simulink model "pendenc"  (Simulink 6.2)
settings: Solver=ode45  StartTime=0.0  StopTime=100.0  RelTol=1e-4
libraries: cstblocks x10, simulink x6
settings Model: Creator=mbarton  LastModifiedBy=mbarton  ExtModeTrigMode=oneshot  ExtModeArmWhenConnect=off  ExtModeAutoUpdateStatusClock=off  BufferReuse=off
settings DataIOCC: LimitDataPoints=off
settings OptimizationCC: BlockReduction=off  BooleanDataType=off  InlineParams=on  InlineInvariantSignals=on  BufferReuse=off
settings HardwareCC: TargetUnknown=on

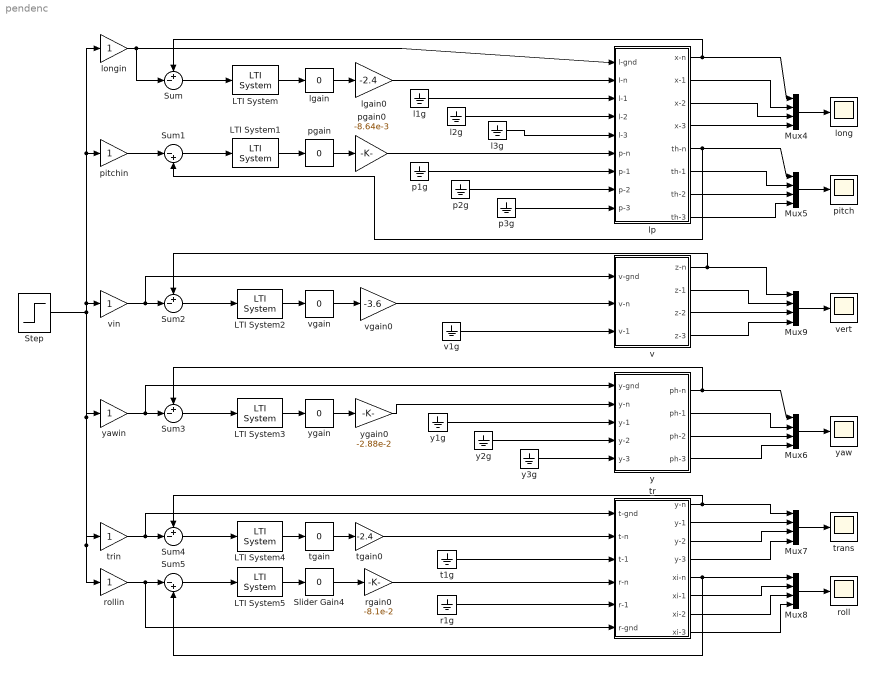
== system pendenc ==
  LTI System : cstblocks/LTI System  sys=ldamp  IC=[]
  LTI System1 : cstblocks/LTI System  sys=pdamp  IC=[]
  LTI System2 : cstblocks/LTI System  sys=vdamp  IC=[]
  LTI System3 : cstblocks/LTI System  sys=ydamp  IC=[]
  LTI System4 : cstblocks/LTI System  sys=tdamp  IC=[]
  LTI System5 : cstblocks/LTI System  sys=rdamp  IC=[]
  Mux{4..9} (6 alike) : Mux
  Slider Gain4 : simulink/Math Operations/Slider Gain  low=0  gain=0  high=2
  Step : Step  Before=1  After=0  SampleTime=0
  Sum{,2..4} (4 alike) : Sum  Inputs=+-|  InputSameDT=on
  Sum1 : Sum  Inputs=|-+  InputSameDT=on
  Sum5 : Sum  Inputs=|-+  InputSameDT=on
  l1g : Ground
  l2g : Ground
  l3g : Ground
  lgain : simulink/Math Operations/Slider Gain  low=0  gain=0  high=2
  lgain0 : Gain  Gain=-2.4
  long : Scope
  longin : Gain
  lp : Subsystem
  p1g : Ground
  p2g : Ground
  p3g : Ground
  pgain : simulink/Math Operations/Slider Gain  low=0  gain=0  high=2
  pgain0 : Gain  Gain=-8.64e-3
  pitch : Scope
  pitchin : Gain
  r1g : Ground
  rgain0 : Gain  Gain=-8.1e-2
  roll : Scope
      settings: YMin=-2  YMax=2
  rollin : Gain
  t1g : Ground
  tgain : simulink/Math Operations/Slider Gain  low=0  gain=0  high=2
  tgain0 : Gain  Gain=-2.4
  tr : Subsystem
  trans : Scope
  trin : Gain
  v : Subsystem
  v1g : Ground
  vert : Scope
      settings: YMin=-2  YMax=2
  vgain : simulink/Math Operations/Slider Gain  low=0  gain=0  high=2
  vgain0 : Gain  Gain=-3.6
  vin : Gain
  y : Subsystem
  y1g : Ground
  y2g : Ground
  y3g : Ground
  yaw : Scope
      settings: YMin=-2  YMax=2
  yawin : Gain
  ygain : simulink/Math Operations/Slider Gain  low=0  gain=0  high=2
  ygain0 : Gain  Gain=-2.88e-2
  wires:
  Step/1 -> pitchin/1, longin/1, vin/1, rollin/1, trin/1, yawin/1
  Mux8/1 -> roll/1
  Mux7/1 -> trans/1
  Mux6/1 -> yaw/1
  Mux9/1 -> vert/1
  Mux5/1 -> pitch/1
  Mux4/1 -> long/1
  lgain0/1 -> lp/2(I-n)
  vgain0/1 -> v/2(v-n)
  ygain0/1 -> y/2(y-n)
  tgain0/1 -> tr/2(t-n)
  rgain0/1 -> tr/4(r-n)
  pgain0/1 -> lp/6(p-n)
  tr/7(xi-2) -> Mux8/3
  tr/6(xi-1) -> Mux8/2
  tr/2(y-1) -> Mux7/2
  y/2(ph-1) -> Mux6/2
  y/3(ph-2) -> Mux6/3
  v/2(z-1) -> Mux9/2
  v/3(z-2) -> Mux9/3
  y/1(ph-n) -> Mux6/1, Sum3/1
  tr/5(xi-n) -> Mux8/1, Sum5/2
  tr/1(y-n) -> Mux7/1, Sum4/1
  lp/5(th-n) -> Sum1/2, Mux5/1
  lp/1(x-n) -> Sum/1, Mux4/1
  lp/2(x-1) -> Mux4/2
  tr/3(y-2) -> Mux7/3
  ygain/1 -> ygain0/1
  vgain/1 -> vgain0/1
  tgain/1 -> tgain0/1
  lgain/1 -> lgain0/1
  pgain/1 -> pgain0/1
  Slider Gain4/1 -> rgain0/1
  LTI System/1 -> lgain/1
  LTI System2/1 -> vgain/1
  Sum1/1 -> LTI System1/1
  LTI System1/1 -> pgain/1
  LTI System3/1 -> ygain/1
  Sum3/1 -> LTI System3/1
  LTI System4/1 -> tgain/1
  Sum4/1 -> LTI System4/1
  LTI System5/1 -> Slider Gain4/1
  Sum5/1 -> LTI System5/1
  v/1(z-n) -> Mux9/1, Sum2/1
  lp/3(x-2) -> Mux4/3
  lp/6(th-1) -> Mux5/2
  v1g/1 -> v/3(v-1)
  y3g/1 -> y/5(y-3)
  t1g/1 -> tr/3(t-1)
  Sum/1 -> LTI System/1
  Sum2/1 -> LTI System2/1
  lp/4(x-3) -> Mux4/4
  lp/7(th-2) -> Mux5/3
  lp/8(th-3) -> Mux5/4
  v/4(z-3) -> Mux9/4
  y/4(ph-3) -> Mux6/4
  tr/4(y-3) -> Mux7/4
  tr/8(xi-3) -> Mux8/4
  rollin/1 -> tr/6(r-gnd), Sum5/1
  trin/1 -> tr/1(t-gnd), Sum4/2
  yawin/1 -> y/1(y-gnd), Sum3/2
  vin/1 -> v/1(v-gnd), Sum2/2
  pitchin/1 -> Sum1/1
  longin/1 -> Sum/2, lp/1(l-gnd)
  l1g/1 -> lp/3(l-1)
  l2g/1 -> lp/4(l-2)
  l3g/1 -> lp/5(l-3)
  p1g/1 -> lp/7(p-1)
  p2g/1 -> lp/8(p-2)
  p3g/1 -> lp/9(p-3)
  y1g/1 -> y/3(y-1)
  y2g/1 -> y/4(y-2)
  r1g/1 -> tr/5(r-1)

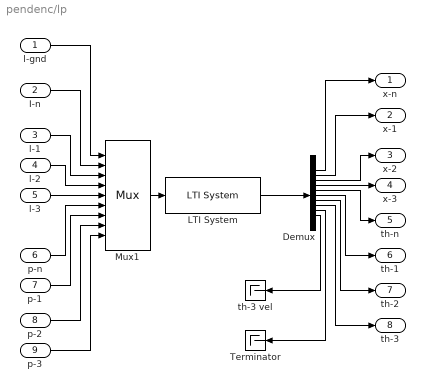
== system pendenc/lp ==
  l-gnd : Inport  Port=1  LatchInput=off
  I-n : Inport  Port=2  LatchInput=off
  l-1 : Inport  Port=3  LatchInput=off
  l-2 : Inport  Port=4  LatchInput=off
  l-3 : Inport  Port=5  LatchInput=off
  p-n : Inport  Port=6  LatchInput=off
  p-1 : Inport  Port=7  LatchInput=off
  p-2 : Inport  Port=8  LatchInput=off
  p-3 : Inport  Port=9  LatchInput=off
  Demux : Demux  Outputs=10
  LTI System : cstblocks/LTI System  sys=lpe  IC=[0]
  Mux1 : Mux  Inputs=9
      settings: DisplayOption=signals
  Terminator : Terminator
  th-3 vel : Terminator
  x-n : Outport
  x-1 : Outport  Port=2
  x-2 : Outport  Port=3
  x-3 : Outport  Port=4
  th-n : Outport  Port=5
  th-1 : Outport  Port=6
  th-2 : Outport  Port=7
  th-3 : Outport  Port=8
  wires:
  Mux1/1 -> LTI System/1
  LTI System/1 -> Demux/1
  Demux/1 -> x-n/1
  Demux/2 -> x-1/1
  Demux/3 -> x-2/1
  Demux/4 -> x-3/1
  Demux/5 -> th-n/1
  Demux/6 -> th-1/1
  Demux/7 -> th-2/1
  Demux/8 -> th-3/1
  l-gnd/1 -> Mux1/1
  I-n/1 -> Mux1/2
  l-1/1 -> Mux1/3
  l-2/1 -> Mux1/4
  l-3/1 -> Mux1/5
  p-n/1 -> Mux1/6
  p-1/1 -> Mux1/7
  p-2/1 -> Mux1/8
  p-3/1 -> Mux1/9
  Demux/9 -> Terminator/1
  Demux/10 -> th-3 vel/1

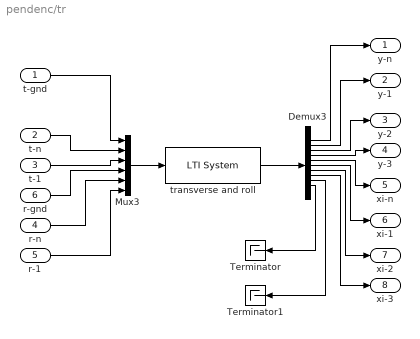
== system pendenc/tr ==
  t-gnd : Inport  Port=1  LatchInput=off
  t-n : Inport  Port=2  LatchInput=off
  t-1 : Inport  Port=3  LatchInput=off
  r-n : Inport  Port=4  LatchInput=off
  r-1 : Inport  Port=5  LatchInput=off
  r-gnd : Inport  Port=6  LatchInput=off
  Demux3 : Demux  Outputs=10
  Mux3 : Mux  Inputs=6
  Terminator : Terminator
  Terminator1 : Terminator
  transverse and roll : cstblocks/LTI System  sys=trer  IC=[0]
  y-n : Outport
  y-1 : Outport  Port=2
  y-2 : Outport  Port=3
  y-3 : Outport  Port=4
  xi-n : Outport  Port=5
  xi-1 : Outport  Port=6
  xi-2 : Outport  Port=7
  xi-3 : Outport  Port=8
  wires:
  Mux3/1 -> transverse and roll/1
  transverse and roll/1 -> Demux3/1
  Demux3/1 -> y-n/1
  Demux3/2 -> y-1/1
  Demux3/3 -> y-2/1
  Demux3/4 -> y-3/1
  Demux3/5 -> xi-n/1
  Demux3/6 -> xi-1/1
  Demux3/7 -> xi-2/1
  Demux3/8 -> xi-3/1
  t-gnd/1 -> Mux3/1
  t-n/1 -> Mux3/2
  t-1/1 -> Mux3/3
  r-1/1 -> Mux3/6
  r-n/1 -> Mux3/5
  r-gnd/1 -> Mux3/4
  Demux3/9 -> Terminator1/1
  Demux3/10 -> Terminator/1

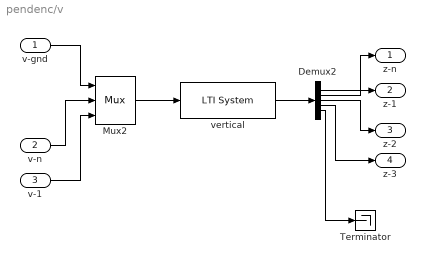
== system pendenc/v ==
  v-gnd : Inport  Port=1  LatchInput=off
  v-n : Inport  Port=2  LatchInput=off
  v-1 : Inport  Port=3  LatchInput=off
  Demux2 : Demux  Outputs=5
  Mux2 : Mux  Inputs=3
      settings: DisplayOption=signals
  Terminator : Terminator
  vertical : cstblocks/LTI System  sys=ve  IC=[0]
  z-n : Outport
  z-1 : Outport  Port=2
  z-2 : Outport  Port=3
  z-3 : Outport  Port=4
  wires:
  Mux2/1 -> vertical/1
  vertical/1 -> Demux2/1
  v-gnd/1 -> Mux2/1
  Demux2/1 -> z-n/1
  Demux2/2 -> z-1/1
  Demux2/3 -> z-2/1
  Demux2/4 -> z-3/1
  v-1/1 -> Mux2/3
  v-n/1 -> Mux2/2
  Demux2/5 -> Terminator/1

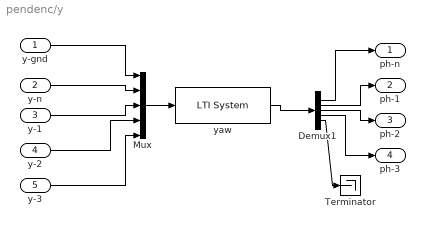
== system pendenc/y ==
  y-gnd : Inport  Port=1  LatchInput=off
  y-n : Inport  Port=2  LatchInput=off
  y-1 : Inport  Port=3  LatchInput=off
  y-2 : Inport  Port=4  LatchInput=off
  y-3 : Inport  Port=5  LatchInput=off
  Demux1 : Demux  Outputs=5
  Mux : Mux  Inputs=5
  Terminator : Terminator
  yaw : cstblocks/LTI System  sys=ye  IC=[0]
  ph-n : Outport
  ph-1 : Outport  Port=2
  ph-2 : Outport  Port=3
  ph-3 : Outport  Port=4
  wires:
  y-gnd/1 -> Mux/1
  Mux/1 -> yaw/1
  yaw/1 -> Demux1/1
  Demux1/1 -> ph-n/1
  Demux1/2 -> ph-1/1
  Demux1/3 -> ph-2/1
  Demux1/4 -> ph-3/1
  y-3/1 -> Mux/5
  y-2/1 -> Mux/4
  y-1/1 -> Mux/3
  y-n/1 -> Mux/2
  Demux1/5 -> Terminator/1
